simulink model "CruiseControl"  (R2020b)
settings: Solver=ode45  StartTime=0.0  StopTime=10.0  RelTol=1e-3
undefined symbols (not defined in the file): Ki, Kp
settings Model: DataDictionary=cruise_control_dd.sldd  Creator=ADMIN  LastModifiedBy=ADMIN

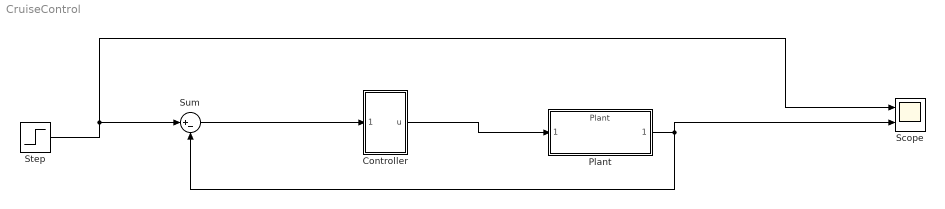
== system CruiseControl ==
  Controller : Subsystem
  Plant : ModelReference  ModelNameDialog=Plant  ModelReferenceVersion=1.6
  Scope : Scope  NumInputPorts=2
  Step : Step  After=40  SampleTime=0
  Sum : Sum  Inputs=|+-
  wires:
  Step/1 -> Scope/1, Sum/1
  Plant/1 -> Sum/2, Scope/2
  Sum/1 -> Controller/1(error)
  Controller/1(u) -> Plant/1

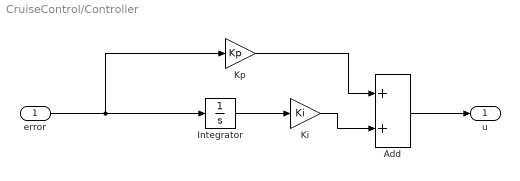
== system CruiseControl/Controller ==
  error : Inport
  Add : Sum
  Integrator : Integrator
  Ki : Gain  Gain=Ki
  Kp : Gain  Gain=Kp
  u : Outport
  wires:
  Integrator/1 -> Ki/1
  Kp/1 -> Add/1
  Ki/1 -> Add/2
  Add/1 -> u/1
  error/1 -> Kp/1, Integrator/1
